simulink model "TwoTanks_FO_R2018a"  (R2018a)
settings: Solver=ode4  StartTime=0.0  StopTime=tfinal  FixedStep=dt  RelTol=1e-3  EnableMultiTasking=on
values from neighbouring files (symbols this model uses):
  a1 = num1/den1    [TwoTanks_FO_main.m]
  a2 = num2/den2    [TwoTanks_FO_main.m]
  a3 = num3/den3    [TwoTanks_FO_main.m]
  a4 = num4/den4    [TwoTanks_FO_main.m]
  Aout1 = pi*(Dout^2)/4    (= 0.00196349540849)    [TwoTanks_FO_main.m]    (also in TwoTanks_NL_main.m)
  Aout2 = Aout1*2/3    (= 0.001308996939)    [TwoTanks_FO_main.m]    (also in TwoTanks_NL_main.m)
  Area1 = pi*D1^2/4    (= 0.0146390957633)    [TwoTanks_FO_main.m]    (also in TwoTanks_NL_main.m)
  Fnom = 30    [TwoTanks_FO_main.m]    (also in TwoTanks_NL_main.m)
  g = 9.81    [TwoTanks_FO_main.m]    (also in TwoTanks_NL_main.m)
  h10 = 0.1    [TwoTanks_FO_main.m]    (also in TwoTanks_NL_main.m)
  H1max = 30*2.54/100    (= 0.762)    [TwoTanks_FO_main.m]    (also in TwoTanks_NL_main.m)
  h20 = 0.1    [TwoTanks_FO_main.m]    (also in TwoTanks_NL_main.m)
  H2max = 0.7    [TwoTanks_FO_main.m]
  K0 = P1(1,3)    [TwoTanks_FO_main.m]
  K1 = P1(1,2)    [TwoTanks_FO_main.m]
  pho = 998.23    [TwoTanks_FO_main.m]    (also in TwoTanks_NL_main.m)
  Qe = pho*Aout1*sqrt(2*g*H1max)    [TwoTanks_FO_main.m]    (also in TwoTanks_NL_main.m)
  R2max = 0.176    [TwoTanks_FO_main.m]
settings Model: Creator=joniram  LastModifiedBy=generic-user
settings DataIOCC: ExternalInput=[limV1F_sup, limV1F_inf, limV2F_sup, limV2F_inf]  LimitDataPoints=on  SaveFormat=Array  SignalLoggingSaveFormat=ModelDataLogs
settings OptimizationCC: ExpressionDepthLimit=2147483647  LifeSpan=inf
settings DebuggingCC: UnderspecifiedInitializationDetection=Classic  MergeDetectMultiDrivingBlocksExec=none  SolverPrmCheckMsg=warning  FcnCallInpInsideContextMsg=warning  StateNameClashWarn=warning  SFUnexpectedBacktrackingDiag=warning  SFNoUnconditionalDefaultTransitionDiag=warning  SFExecutionAtInitializationDiag=none
settings HardwareCC: ProdBitPerPointer=32  ProdBitPerSizeT=32  ProdBitPerPtrDiffT=32  ProdLargestAtomicFloat=None  ProdIntDivRoundTo=Undefined  ProdEndianess=Unspecified  ProdWordSize=32  ProdHWDeviceType=32-bit Generic
settings ModelReferenceCC: PropagateSignalLabelsOutOfModel=off
settings CodeAppCC: StateflowObjectComments=on
settings GRTTargetCC: TargetLangStandard=C89/C90 (ANSI)  GeneratePreprocessorConditionals=Disable all  CombineOutputUpdateFcns=off  GRTInterface=on
settings ConfigComp: CovMetricSettings=dw  CovHtmlReporting=on  CovSaveCumulativeToWorkspaceVar=on  CovSaveSingleToWorkspaceVar=on  CovExternalEMLEnable=off

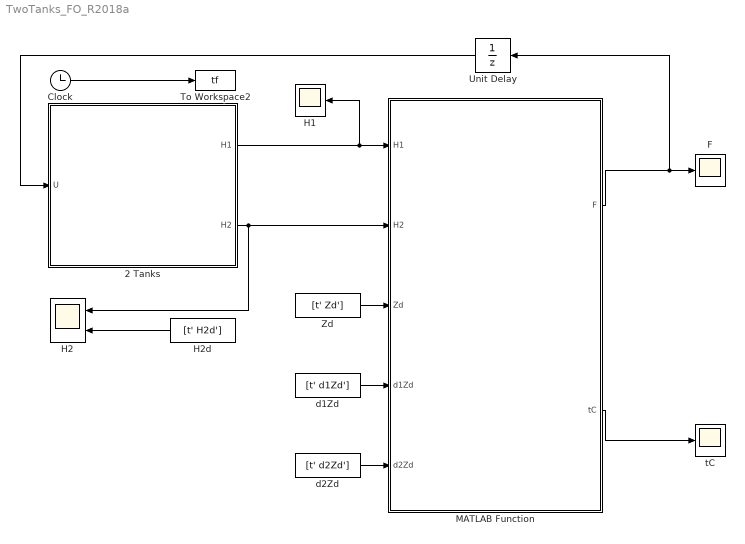
== system TwoTanks_FO_R2018a ==
  2 Tanks : Subsystem
  Clock : Clock
  F : Scope
  H1 : Scope
  H2 : Scope  NumInputPorts=2
  H2d : FromWorkspace  VariableName=[t' H2d']  SampleTime=0  OutputAfterFinalValue=Holding final value
  MATLAB Function : MATLAB Function  TreatAsAtomicUnit=on
  To Workspace2 : ToWorkspace  VariableName=tf  SampleTime=-1
  Unit Delay : UnitDelay  SampleTime=-1
  Zd : FromWorkspace  VariableName=[t' Zd']  SampleTime=0  OutputAfterFinalValue=Holding final value
  d1Zd : FromWorkspace  VariableName=[t' d1Zd']  SampleTime=0  OutputAfterFinalValue=Holding final value
  d2Zd : FromWorkspace  VariableName=[t' d2Zd']  SampleTime=0  OutputAfterFinalValue=Holding final value
  tC : Scope
  wires:
  2 Tanks/2(H2) -> MATLAB Function/2(H2), H2/1
  2 Tanks/1(H1) -> H1/1, MATLAB Function/1(H1)
  d2Zd/1 -> MATLAB Function/5(d2Zd)
  Zd/1 -> MATLAB Function/3(Zd)
  d1Zd/1 -> MATLAB Function/4(d1Zd)
  MATLAB Function/1(F) -> Unit Delay/1, F/1
  MATLAB Function/2(tC) -> tC/1
  Unit Delay/1 -> 2 Tanks/1(U)
  H2d/1 -> H2/2
  Clock/1 -> To Workspace2/1

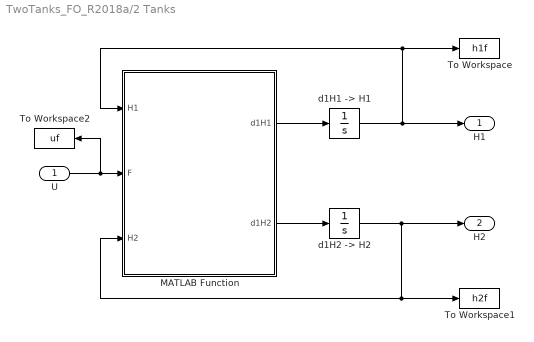
== system TwoTanks_FO_R2018a/2 Tanks ==
  U : Inport
  MATLAB Function : MATLAB Function  TreatAsAtomicUnit=on
  To Workspace : ToWorkspace  VariableName=h1f  SampleTime=-1
  To Workspace1 : ToWorkspace  VariableName=h2f  SampleTime=-1
  To Workspace2 : ToWorkspace  VariableName=uf  SampleTime=-1
  "d1H1 -> H1" : Integrator  InitialCondition=h10  LimitOutput=on  UpperSaturationLimit=H1max  LowerSaturationLimit=0
  "d1H2 -> H2" : Integrator  InitialCondition=h20  LimitOutput=on  UpperSaturationLimit=H2max  LowerSaturationLimit=0
  H1 : Outport
  H2 : Outport  Port=2
  wires:
  MATLAB Function/1(d1H1) -> "d1H1 -> H1"/1
  "d1H1 -> H1"/1 -> H1/1, To Workspace/1, MATLAB Function/1(H1)
  MATLAB Function/2(d1H2) -> "d1H2 -> H2"/1
  U/1 -> To Workspace2/1, MATLAB Function/2(F)
  "d1H2 -> H2"/1 -> H2/1, To Workspace1/1, MATLAB Function/3(H2)

== matlab function TwoTanks_FO_R2018a/2 Tanks/MATLAB Function ==
  data: H1 input; F input; d1H1 output; H2 input; d1H2 output; pho parameter; Fnom parameter; Area1 parameter; Aout2 parameter; H2max parameter; Aout1 parameter; g parameter; Qe parameter; R2max parameter
function [d1H1, d1H2] = TwoTanks(H1, F, H2, pho, Fnom, Area1, Aout2, H2max, Aout1, g, Qe, R2max)

  % Parametros - d1H1
    num1 = Qe;
    den1 = pho*Area1*(Fnom);
    num2 = Aout1*sqrt(2*g);
    den2 = Area1;
  
  % Parametros - d1H2
    num3 = Aout1*sqrt(2*g)*H2max^2;
    den3 = pi*R2max^2;
    num4 = Aout2*sqrt(2*g)*H2max^2;
    den4 = pi*R2max^2;
  
  % Sistema Dinâmico
    d1H1 = (num1/den1)*(F) - (num2/den2)*sqrt(H1);
    
    d1H2 = (num3/den3)*(sqrt(H1)/(H2^2)) - (num4/den4)*(1/(H2^1.5));

== matlab function TwoTanks_FO_R2018a/MATLAB Function ==
  data: F output; tC output; H1 input; H2 input; K1 parameter; K0 parameter; Zd input; d1Zd input; d2Zd input; a1 parameter; a2 parameter; a3 parameter; a4 parameter
function [F, tC]  = Controle_Flatness(H1, H2, K1, K0, Zd, d1Zd, d2Zd, a1, a2, a3, a4)
 
  % Gerando Z e d1Z
    Z = H2;
    d1Z = a3*(sqrt(H1)/(H2^2)) - a4/(H2^1.5);
    
  % Termo de Correção em Malha Fechada
    tC = d2Zd - K1*(d1Z - d1Zd) - K0*(Z - Zd); 
    
  % Gerando a expressão final para os controladores
    F = ((2*Z^(5/2)*a4 + 2*Z^4*d1Z)/(a1*a3^2))*tC + (a4^2*d1Z + 4*H2^3*d1Z^3 + 5*Z^(3/2)*a4*d1Z^2 + a2*a3^2*((Z*(a4 + Z^(3/2)*d1Z)^2)/a3^2)^(1/2))/(a1*a3^2);
    
 
  % Saturação dos Sinais de Controle
    limF_sup = 200; limF_inf = 10;
    F = min(limF_sup, max(limF_inf, F));
